simulink model "sim_battery_pack_simulink_with_EV_Load"  (R2021b)
settings: Solver=FixedStepAuto  StartTime=0.0  StopTime=3460.480  FixedStep=0.01  RelTol=1e-3
values from neighbouring files (symbols this model uses):
  Af = 1.4*1.6    (= 2.24)    [battery_pack_init_18_11.m]
  b = 0.002    [battery_pack_init_18_11.m]
  Batt_Eff = .98    (= 0.98)    [battery_pack_init_18_11.m]
  Batt_Ene_Cap = 7.37    [battery_pack_init_18_11.m]
  cd = 0.45    [battery_pack_init_18_11.m]
  dt = 0.01    [battery_pack_init_18_11.m]
  g = 9.81    [battery_pack_init_18_11.m]
  Gr = 5.75*.85    (= 4.8875)    [battery_pack_init_18_11.m]
  Grade = 7    [battery_pack_init_18_11.m]
  Ini_SOC = 100    [battery_pack_init_18_11.m]
  kappa = 0.1    [battery_pack_init_18_11.m]
  M = M_k+M_P    (= 445)    [battery_pack_init_18_11.m]
  M_Trq = T_m    [battery_pack_init_18_11.m]
  M_w = w_m    [battery_pack_init_18_11.m]
  Mot_Eff = .9    (= 0.9)    [battery_pack_init_18_11.m]
  mu = 0.016    [battery_pack_init_18_11.m]
  Np = 7    [battery_pack_init_18_11.m]
  Ns = 12    [battery_pack_init_18_11.m]
  Qgain = 1    [battery_pack_init_18_11.m]
  R0 = zeros(numpoles,1)    [battery_pack_init_18_11.m]
  R0Param = getParamESC('R0Param',T,cell_model)    [battery_pack_init_18_11.m]
  R_w = .3048/2    (= 0.1524)    [battery_pack_init_18_11.m]
  Re_spe_max = 50*5/18    (= 13.8888888889)    [battery_pack_init_18_11.m]
  Re_spe_min = 0*5/18    (= 0)    [battery_pack_init_18_11.m]
  rho = 1.225    [battery_pack_init_18_11.m]
  rt = .0008    (= 0.0008)    [battery_pack_init_18_11.m]
  T = 40    [battery_pack_init_18_11.m]
  T_MIDC = T_MIDC(1:72)    [battery_pack_init_18_11.m]
  Trans_Eff = .95    (= 0.95)    [battery_pack_init_18_11.m]
  V_MIDC = V_MIDC(1:72)    [battery_pack_init_18_11.m]
  Z0 = 0.75 + (1-0.75).*rand(1,Np)    [battery_pack_init_18_11.m]
undefined symbols (not defined in the file or in its folder): cell_model, FLbattery, gain, iload, sigbuilder_block, VMIDC
libraries: simulink x16, autolibshared x2, slpidlib x1, simulink_extras x1
(part 1 of 17)
settings Model: Creator=User  LastModifiedBy=adhip
settings SolverCC: AlgebraicLoopSolver=TrustRegion

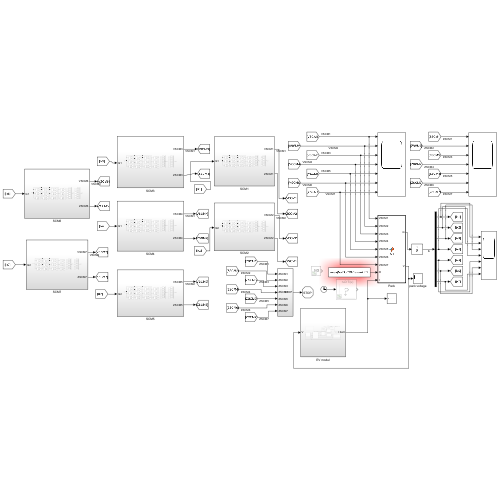
[thumbnail: Simulink's stored preview of the top-level diagram]
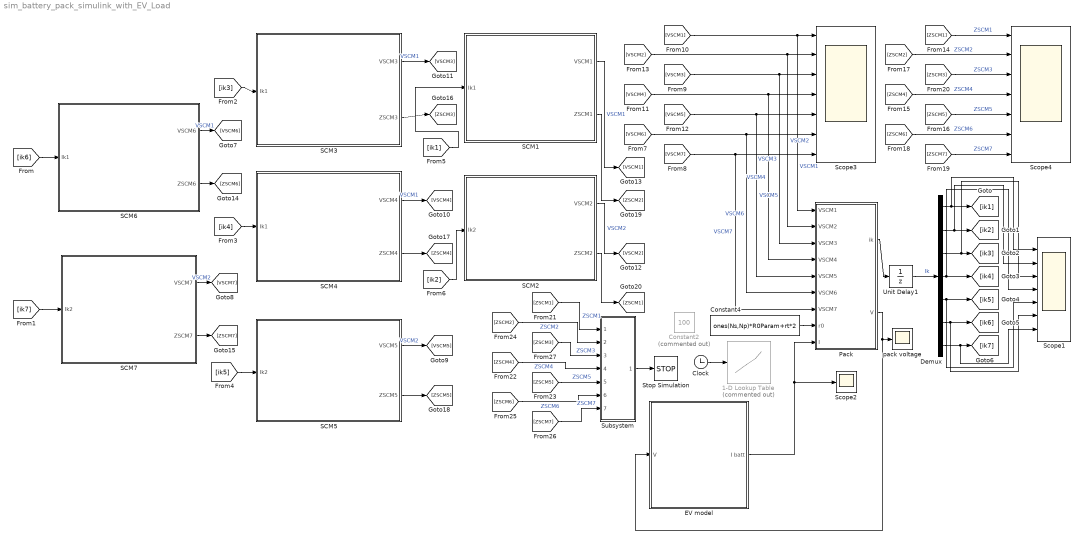
== system sim_battery_pack_simulink_with_EV_Load ==
  1-D Lookup Table : Lookup_n-D  Commented=on  NumberOfTableDimensions=1  BreakpointsForDimension1=0:0.01:3460.480  Table=iload  InternalRulePriority=Speed  RndMeth=Simplest  InputSameDT=on
  Clock : Clock
  Constant2 : Constant  Commented=on  Value=100
  Constant4 : Constant  Value=ones(Ns,Np)*R0Param+rt*2
  Demux : Demux  Outputs=7
  EV model : Subsystem
  Pack : MATLAB Function  TreatAsAtomicUnit=on
  SCM1 : Subsystem
  SCM2 : Subsystem
  SCM3 : Subsystem
  SCM4 : Subsystem
  SCM5 : Subsystem
  SCM6 : Subsystem
  SCM7 : Subsystem
  Scope1 : Scope  NumInputPorts=7
  Scope2 : Scope
  Scope3 : Scope  NumInputPorts=7
  Scope4 : Scope  NumInputPorts=7
  Stop Simulation : Stop
  Subsystem : Subsystem
  Unit Delay1 : UnitDelay  SampleTime=-1  HasFrameUpgradeWarning=on
  pack voltage : Scope
  wires:
  EV model/1(I batt) -> Pack/9(I), Scope2/1
  [VSCM1] -> Pack/1(VSCM1), Scope3/1  "VSCM1"
  [VSCM2] -> Scope3/2, Pack/2(VSCM2)  "VSCM2"
  Pack/1(ik) -> Unit Delay1/1
  Unit Delay1/1 -> Demux/1  "Ik"
  Constant4/1 -> Pack/8(r0)
  Clock/1 -> 1-D Lookup Table/1
  [VSCM3] -> Scope3/3, Pack/3(VSCM3)  "VSCM3"
  [VSCM4] -> Pack/4(VSCM4), Scope3/4  "VSCM4"
  [VSCM5] -> Pack/5(VSCM5), Scope3/5  "VSCM5"
  [VSCM6] -> Pack/6(VSCM6), Scope3/6  "VSCM6"
  [VSCM7] -> Scope3/7, Pack/7(VSCM7)  "VSCM7"
  [ik7] -> SCM7/1(Ik2)
  [ik6] -> SCM6/1(Ik1)
  [ik3] -> SCM3/1(Ik1)
  [ik4] -> SCM4/1(Ik1)
  [ik5] -> SCM5/1(Ik2)
  [ik2] -> SCM2/1(Ik2)
  [ik1] -> SCM1/1(Ik1)
  Demux/1 -> Scope1/1, [ik1]
  Demux/2 -> [ik2], Scope1/2
  Demux/3 -> Scope1/3, [ik3]
  Demux/4 -> [ik4], Scope1/4
  Demux/5 -> [ik5], Scope1/5
  Demux/6 -> [ik6], Scope1/6
  Demux/7 -> Scope1/7, [ik7]
  SCM6/1(VSCM6) -> [VSCM6]  "VSCM1"
  SCM7/1(VSCM7) -> [VSCM7]  "VSCM2"
  SCM1/1(VSCM1) -> [VSCM1]  "VSCM1"
  SCM2/1(VSCM2) -> [VSCM2]  "VSCM2"
  SCM5/1(VSCM5) -> [VSCM5]  "VSCM2"
  SCM4/1(VSCM4) -> [VSCM4]  "VSCM1"
  SCM3/1(VSCM3) -> [VSCM3]  "VSCM1"
  Pack/2(V) -> pack voltage/1, EV model/1(V)
  SCM6/2(ZSCM6) -> [ZSCM6]
  SCM7/2(ZSCM7) -> [ZSCM7]
  SCM3/2(ZSCM3) -> [ZSCM3]
  SCM4/2(ZSCM4) -> [ZSCM4]
  SCM5/2(ZSCM5) -> [ZSCM5]
  SCM1/2(ZSCM1) -> [ZSCM2]
  SCM2/2(ZSCM2) -> [ZSCM1]
  [ZSCM7] -> Scope4/7  "ZSCM7"
  [ZSCM6] -> Scope4/6  "ZSCM6"
  [ZSCM5] -> Scope4/5  "ZSCM5"
  [ZSCM4] -> Scope4/4  "ZSCM4"
  [ZSCM3] -> Scope4/3  "ZSCM3"
  [ZSCM2] -> Scope4/2  "ZSCM2"
  [ZSCM1] -> Scope4/1  "ZSCM1"
  [ZSCM2] -> Subsystem/2(ZSCM2)  "ZSCM2"
  [ZSCM4] -> Subsystem/4(ZSCM4)  "ZSCM4"
  [ZSCM6] -> Subsystem/6(ZSCM6)  "ZSCM6"
  [ZSCM1] -> Subsystem/1(ZSCM1)  "ZSCM1"
  [ZSCM3] -> Subsystem/3(ZSCM3)  "ZSCM3"
  [ZSCM5] -> Subsystem/5(ZSCM5)  "ZSCM5"
  [ZSCM7] -> Subsystem/7(ZSCM7)  "ZSCM7"
  Subsystem/1(STOP) -> Stop Simulation/1

== system sim_battery_pack_simulink_with_EV_Load/EV model ==
  V : Inport
  Battery1 : Subsystem
      settings: PortSchema="{\"entries\":[{\"content\":{\"sides\":[{\"content\":{\"connectorIds\":[\"Out4\",\"In1\"]},\"type\":\"ConnectorPlacement.EquallySpacedRectSide\",\"uuid\":\"95f9873b-fe01-4ff7-a5ab-aada3bc95a03\"},{\"content\":{\"connectorIds\":[\"Out1\",\"In2\",\"Out2\",\"Out3\"],\"side\":\"RIGHT\"},\"type\":\"ConnectorPlacement.EquallySpacedRectSide\",\"uuid\":\"b4897c1e-778c-4bc7-a7f1-163b7f4cdad4\"},{\"content\":{\"connectorIds\":[],\"side\":\"TOP\"},\"type\":\"ConnectorPlacement.EquallySpacedRectSide\",\"uuid\":\"a4f74249-cbee-46b9-95a1-ffe2d651d1aa\"}]},\"type\":\"ConnectorPlacement.EquallySpacedConnector\",\"uuid\":\"65519a53-4300-47bd-84a6-9cdab8c1658d\"}],\"packageUris\":[\"http://schema.mathworks.com/mf0/Connector/R2020b\"],\"version\":\"1.0\"}"
  Constant3 : Constant  Value=7.37
  Constant4 : Constant
  Controller : Subsystem
      settings: PortSchema="{\"entries\":[{\"content\":{\"sides\":[{\"content\":{\"connectorIds\":[\"In1\",\"In2\",\"In3\"]},\"type\":\"ConnectorPlacement.EquallySpacedRectSide\",\"uuid\":\"7181f2fb-814d-454b-bbdd-5a6429464cde\"},{\"content\":{\"connectorIds\":[\"Out1\",\"In6\",\"Out2\"],\"side\":\"RIGHT\"},\"type\":\"ConnectorPlacement.EquallySpacedRectSide\",\"uuid\":\"9f09df5c-a21b-4dbe-b9f4-fd639a3fc7b6\"},{\"content\":{\"connectorIds\":[\"In4\",\"In5\"],\"side\":\"TOP\"},\"type\":\"ConnectorPlacement.EquallySpacedRectSide\",\"uuid\":\"cea066f6-5d29-4bfe-a52b-88d077042081\"}]},\"type\":\"ConnectorPlacement.EquallySpacedConnector\",\"uuid\":\"89d9cb73-964c-472c-86a0-f36e993decee\"}],\"packageUris\":[\"http://schema.mathworks.com/mf0/Connector/R2020b\"],\"version\":\"1.0\"}"
  Display2 : Display
  Divide : Product  Inputs=*/
  Driver : Subsystem
  Motor : Subsystem
  Product1 : Product
  Scope : Scope
  Scope1 : Scope  NumInputPorts=2
  Subtract : Sum  Inputs=+-
  Transmission : Subsystem
      settings: PortSchema="{\"entries\":[{\"content\":{\"sides\":[{\"content\":{\"connectorIds\":[\"In1\",\"Out2\"]},\"type\":\"ConnectorPlacement.EquallySpacedRectSide\",\"uuid\":\"6a60ea79-1d6a-43be-8c6e-faa96b9426ae\"},{\"content\":{\"connectorIds\":[\"Out1\",\"In2\"],\"side\":\"RIGHT\"},\"type\":\"ConnectorPlacement.EquallySpacedRectSide\",\"uuid\":\"ce7e119a-d2f4-42be-b472-f935cef86375\"},{\"content\":{\"connectorIds\":[],\"side\":\"TOP\"},\"type\":\"ConnectorPlacement.EquallySpacedRectSide\",\"uuid\":\"7967fcd3-5be4-4a26-8ccb-3cce446b495a\"}]},\"type\":\"ConnectorPlacement.EquallySpacedConnector\",\"uuid\":\"10659099-893a-4c78-98f4-a4e8ec8b982a\"}],\"packageUris\":[\"http://schema.mathworks.com/mf0/Connector/R2020b\"],\"version\":\"1.0\"}"
  Vehicle Dynamics : Subsystem
      settings: PortSchema="{\"entries\":[{\"content\":{\"sides\":[{\"content\":{\"connectorIds\":[\"In1\",\"Out3\",\"Out4\",\"In2\"]},\"type\":\"ConnectorPlacement.EquallySpacedRectSide\",\"uuid\":\"6a60ea79-1d6a-43be-8c6e-faa96b9426ae\"},{\"content\":{\"connectorIds\":[\"Out1\"],\"side\":\"RIGHT\"},\"type\":\"ConnectorPlacement.EquallySpacedRectSide\",\"uuid\":\"ce7e119a-d2f4-42be-b472-f935cef86375\"},{\"content\":{\"connectorIds\":[\"Out2\"],\"side\":\"TOP\"},\"type\":\"ConnectorPlacement.EquallySpacedRectSide\",\"uuid\":\"7967fcd3-5be4-4a26-8ccb-3cce446b495a\"}]},\"type\":\"ConnectorPlacement.EquallySpacedConnector\",\"uuid\":\"10659099-893a-4c78-98f4-a4e8ec8b982a\"}],\"packageUris\":[\"http://schema.mathworks.com/mf0/Connector/R2020b\"],\"version\":\"1.0\"}"
  Vehicle Monitoring : Subsystem  Commented=on
  km : Display
  kwhr/km : Display
  I batt : Outport
  tag scope: Soc=global
  wires:
  Product1/1 -> Divide/1
  Battery1/1(SOC) -> [Soc], Scope/1, Display2/1, Subtract/2
  Controller/1(TrqCmd) -> Motor/1(TrqCmd)
  Subtract/1 -> Product1/2
  Constant4/1 -> Subtract/1
  Motor/2(Mtr_trq) -> Transmission/1(MtrTrq)
  Vehicle Dynamics/4(VKm/h) -> Scope1/2
  Battery1/3(Regen_Pow_Lim) -> Controller/5(Regen_Lim)
  Divide/1 -> kwhr/km/1
  Driver/3(Vref) -> Scope1/1
  Driver/2(DecelCmd) -> Controller/2(Brake)
  Motor/1(Batt_Pow_Cons) -> Battery1/1(Battery power)
  Vehicle Dynamics/2(Dis) -> Divide/2, km/1
  Vehicle Dynamics/1(VehSpd) -> Controller/3(VehSpd), Driver/1(VelFdbk)
  Battery1/2(Draw_Pow_Lim) -> Controller/4(Draw_Lim)
  Transmission/1(AxleTrq) -> Vehicle Dynamics/1(AxleTrq)
  Controller/2(BrkForce) -> Vehicle Dynamics/2(BrakeForce)
  Driver/1(AccelCmd) -> Controller/1(AccelCmd)
  Transmission/2(MtrSpd) -> Controller/6(MtrSpd), Motor/2(MtrSpd)
  Vehicle Dynamics/3(AxleSpd) -> Transmission/2(AxleSpd)
  Constant3/1 -> Product1/1
  Battery1/4(I batt) -> I batt/1
  V/1 -> Battery1/2(V)

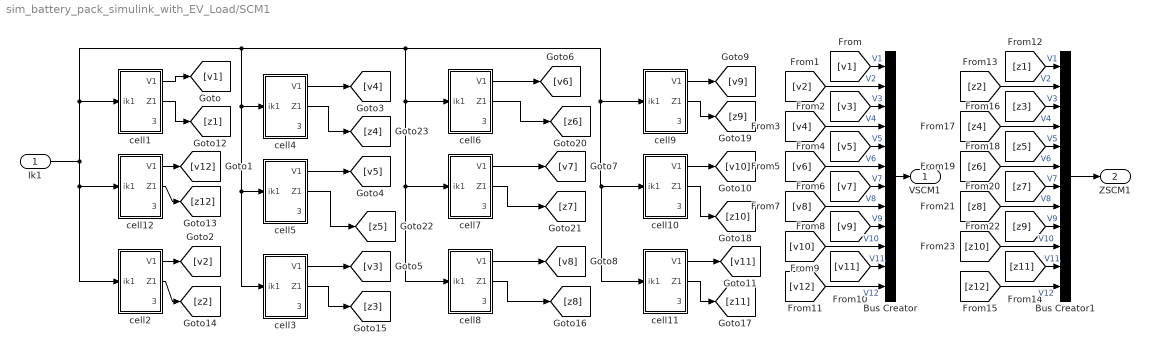
== system sim_battery_pack_simulink_with_EV_Load/SCM1 ==
  Ik1 : Inport
  Bus Creator : BusCreator  Inputs=12
  Bus Creator1 : BusCreator  Inputs=12
  cell1 : Subsystem
  cell10 : Subsystem
  cell11 : Subsystem
  cell12 : Subsystem
  cell2 : Subsystem
  cell3 : Subsystem
  cell4 : Subsystem
  cell5 : Subsystem
  cell6 : Subsystem
  cell7 : Subsystem
  cell8 : Subsystem
  cell9 : Subsystem
  VSCM1 : Outport
  ZSCM1 : Outport  Port=2
  wires:
  cell11/1(V1) -> [v11]
  cell8/1(V1) -> [v8]
  cell2/1(V1) -> [v2]
  cell1/1(V1) -> [v1]
  cell12/1(V1) -> [v12]
  cell7/1(V1) -> [v7]
  cell10/1(V1) -> [v10]
  Ik1/1 -> cell2/1(ik1), cell12/1(ik1), cell1/1(ik1), cell9/1(ik1), cell11/1(ik1), cell10/1(ik1), cell6/1(ik1), cell8/1(ik1), cell7/1(ik1), cell4/1(ik1), cell5/1(ik1), cell3/1(ik1)
  [v1] -> Bus Creator/1  "V1"
  [v2] -> Bus Creator/2  "V2"
  cell4/1(V1) -> [v4]
  cell5/1(V1) -> [v5]
  cell3/1(V1) -> [v3]
  cell6/1(V1) -> [v6]
  cell9/1(V1) -> [v9]
  [v3] -> Bus Creator/3  "V3"
  [v4] -> Bus Creator/4  "V4"
  [v5] -> Bus Creator/5  "V5"
  [v6] -> Bus Creator/6  "V6"
  [v7] -> Bus Creator/7  "V7"
  [v8] -> Bus Creator/8  "V8"
  [v9] -> Bus Creator/9  "V9"
  [v10] -> Bus Creator/10  "V10"
  [v11] -> Bus Creator/11  "V11"
  [v12] -> Bus Creator/12  "V12"
  Bus Creator/1 -> VSCM1/1
  cell1/2(Z1) -> [z1]
  cell12/2(Z1) -> [z12]
  cell2/2(Z1) -> [z2]
  cell8/2(Z1) -> [z8]
  cell11/2(Z1) -> [z11]
  cell10/2(Z1) -> [z10]
  cell9/2(Z1) -> [z9]
  cell6/2(Z1) -> [z6]
  cell7/2(Z1) -> [z7]
  cell3/2(Z1) -> [z3]
  cell5/2(Z1) -> [z5]
  cell4/2(Z1) -> [z4]
  Bus Creator1/1 -> ZSCM1/1
  [z12] -> Bus Creator1/12  "V12"
  [z11] -> Bus Creator1/11  "V11"
  [z10] -> Bus Creator1/10  "V10"
  [z9] -> Bus Creator1/9  "V9"
  [z8] -> Bus Creator1/8  "V8"
  [z7] -> Bus Creator1/7  "V7"
  [z6] -> Bus Creator1/6  "V6"
  [z5] -> Bus Creator1/5  "V5"
  [z4] -> Bus Creator1/4  "V4"
  [z3] -> Bus Creator1/3  "V3"
  [z2] -> Bus Creator1/2  "V2"
  [z1] -> Bus Creator1/1  "V1"

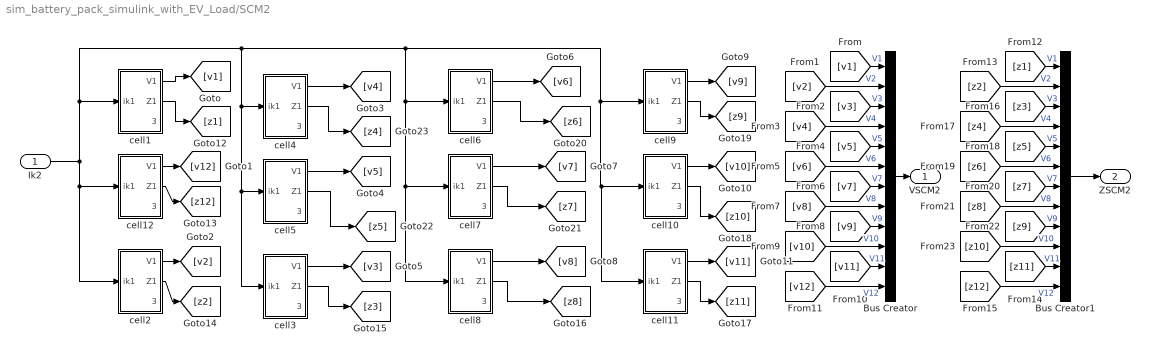
== system sim_battery_pack_simulink_with_EV_Load/SCM2 ==
  Ik2 : Inport
  Bus Creator : BusCreator  Inputs=12
  Bus Creator1 : BusCreator  Inputs=12
  cell1 : Subsystem
  cell10 : Subsystem
  cell11 : Subsystem
  cell12 : Subsystem
  cell2 : Subsystem
  cell3 : Subsystem
  cell4 : Subsystem
  cell5 : Subsystem
  cell6 : Subsystem
  cell7 : Subsystem
  cell8 : Subsystem
  cell9 : Subsystem
  VSCM2 : Outport
  ZSCM2 : Outport  Port=2
  wires:
  [z1] -> Bus Creator1/1  "V1"
  [z2] -> Bus Creator1/2  "V2"
  [z3] -> Bus Creator1/3  "V3"
  [z4] -> Bus Creator1/4  "V4"
  [z5] -> Bus Creator1/5  "V5"
  [z6] -> Bus Creator1/6  "V6"
  [z7] -> Bus Creator1/7  "V7"
  [z8] -> Bus Creator1/8  "V8"
  [z9] -> Bus Creator1/9  "V9"
  [z10] -> Bus Creator1/10  "V10"
  [z11] -> Bus Creator1/11  "V11"
  [z12] -> Bus Creator1/12  "V12"
  Bus Creator1/1 -> ZSCM2/1
  cell4/2(Z1) -> [z4]
  cell5/2(Z1) -> [z5]
  cell3/2(Z1) -> [z3]
  cell7/2(Z1) -> [z7]
  cell6/2(Z1) -> [z6]
  cell9/2(Z1) -> [z9]
  cell10/2(Z1) -> [z10]
  cell11/2(Z1) -> [z11]
  cell8/2(Z1) -> [z8]
  cell2/2(Z1) -> [z2]
  cell12/2(Z1) -> [z12]
  cell1/2(Z1) -> [z1]
  Bus Creator/1 -> VSCM2/1
  [v12] -> Bus Creator/12  "V12"
  [v11] -> Bus Creator/11  "V11"
  [v10] -> Bus Creator/10  "V10"
  [v9] -> Bus Creator/9  "V9"
  [v8] -> Bus Creator/8  "V8"
  [v7] -> Bus Creator/7  "V7"
  [v6] -> Bus Creator/6  "V6"
  [v5] -> Bus Creator/5  "V5"
  [v4] -> Bus Creator/4  "V4"
  [v3] -> Bus Creator/3  "V3"
  cell9/1(V1) -> [v9]
  cell6/1(V1) -> [v6]
  cell3/1(V1) -> [v3]
  cell5/1(V1) -> [v5]
  cell4/1(V1) -> [v4]
  [v2] -> Bus Creator/2  "V2"
  [v1] -> Bus Creator/1  "V1"
  Ik2/1 -> cell3/1(ik1), cell5/1(ik1), cell4/1(ik1), cell7/1(ik1), cell8/1(ik1), cell6/1(ik1), cell10/1(ik1), cell11/1(ik1), cell9/1(ik1), cell1/1(ik1), cell12/1(ik1), cell2/1(ik1)
  cell10/1(V1) -> [v10]
  cell7/1(V1) -> [v7]
  cell12/1(V1) -> [v12]
  cell1/1(V1) -> [v1]
  cell2/1(V1) -> [v2]
  cell8/1(V1) -> [v8]
  cell11/1(V1) -> [v11]

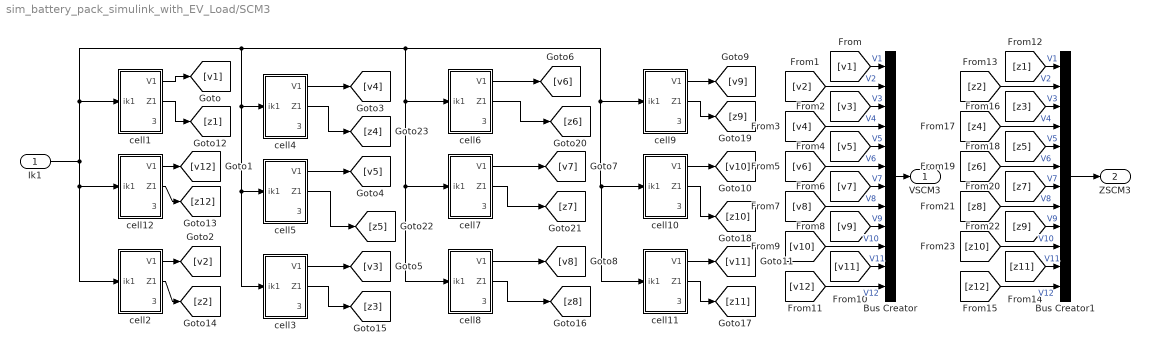
== system sim_battery_pack_simulink_with_EV_Load/SCM3 ==
  Ik1 : Inport
  Bus Creator : BusCreator  Inputs=12
  Bus Creator1 : BusCreator  Inputs=12
  cell1 : Subsystem
  cell10 : Subsystem
  cell11 : Subsystem
  cell12 : Subsystem
  cell2 : Subsystem
  cell3 : Subsystem
  cell4 : Subsystem
  cell5 : Subsystem
  cell6 : Subsystem
  cell7 : Subsystem
  cell8 : Subsystem
  cell9 : Subsystem
  VSCM3 : Outport
  ZSCM3 : Outport  Port=2
  wires:
  cell11/1(V1) -> [v11]
  cell8/1(V1) -> [v8]
  cell2/1(V1) -> [v2]
  cell1/1(V1) -> [v1]
  cell12/1(V1) -> [v12]
  cell7/1(V1) -> [v7]
  cell10/1(V1) -> [v10]
  Ik1/1 -> cell2/1(ik1), cell12/1(ik1), cell1/1(ik1), cell9/1(ik1), cell11/1(ik1), cell10/1(ik1), cell6/1(ik1), cell8/1(ik1), cell7/1(ik1), cell4/1(ik1), cell5/1(ik1), cell3/1(ik1)
  [v1] -> Bus Creator/1  "V1"
  [v2] -> Bus Creator/2  "V2"
  cell4/1(V1) -> [v4]
  cell5/1(V1) -> [v5]
  cell3/1(V1) -> [v3]
  cell6/1(V1) -> [v6]
  cell9/1(V1) -> [v9]
  [v3] -> Bus Creator/3  "V3"
  [v4] -> Bus Creator/4  "V4"
  [v5] -> Bus Creator/5  "V5"
  [v6] -> Bus Creator/6  "V6"
  [v7] -> Bus Creator/7  "V7"
  [v8] -> Bus Creator/8  "V8"
  [v9] -> Bus Creator/9  "V9"
  [v10] -> Bus Creator/10  "V10"
  [v11] -> Bus Creator/11  "V11"
  [v12] -> Bus Creator/12  "V12"
  Bus Creator/1 -> VSCM3/1
  cell1/2(Z1) -> [z1]
  cell12/2(Z1) -> [z12]
  cell2/2(Z1) -> [z2]
  cell8/2(Z1) -> [z8]
  cell11/2(Z1) -> [z11]
  cell10/2(Z1) -> [z10]
  cell9/2(Z1) -> [z9]
  cell6/2(Z1) -> [z6]
  cell7/2(Z1) -> [z7]
  cell3/2(Z1) -> [z3]
  cell5/2(Z1) -> [z5]
  cell4/2(Z1) -> [z4]
  Bus Creator1/1 -> ZSCM3/1
  [z12] -> Bus Creator1/12  "V12"
  [z11] -> Bus Creator1/11  "V11"
  [z10] -> Bus Creator1/10  "V10"
  [z9] -> Bus Creator1/9  "V9"
  [z8] -> Bus Creator1/8  "V8"
  [z7] -> Bus Creator1/7  "V7"
  [z6] -> Bus Creator1/6  "V6"
  [z5] -> Bus Creator1/5  "V5"
  [z4] -> Bus Creator1/4  "V4"
  [z3] -> Bus Creator1/3  "V3"
  [z2] -> Bus Creator1/2  "V2"
  [z1] -> Bus Creator1/1  "V1"

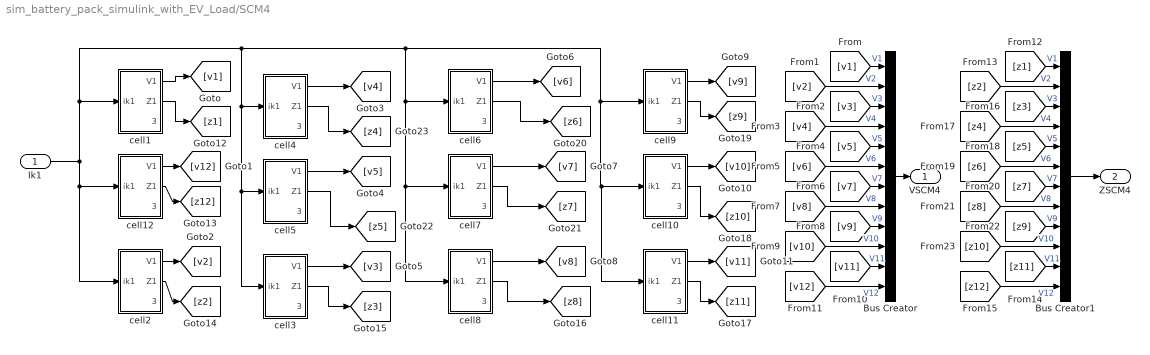
== system sim_battery_pack_simulink_with_EV_Load/SCM4 ==
  Ik1 : Inport
  Bus Creator : BusCreator  Inputs=12
  Bus Creator1 : BusCreator  Inputs=12
  cell1 : Subsystem
  cell10 : Subsystem
  cell11 : Subsystem
  cell12 : Subsystem
  cell2 : Subsystem
  cell3 : Subsystem
  cell4 : Subsystem
  cell5 : Subsystem
  cell6 : Subsystem
  cell7 : Subsystem
  cell8 : Subsystem
  cell9 : Subsystem
  VSCM4 : Outport
  ZSCM4 : Outport  Port=2
  wires:
  [z1] -> Bus Creator1/1  "V1"
  [z2] -> Bus Creator1/2  "V2"
  [z3] -> Bus Creator1/3  "V3"
  [z4] -> Bus Creator1/4  "V4"
  [z5] -> Bus Creator1/5  "V5"
  [z6] -> Bus Creator1/6  "V6"
  [z7] -> Bus Creator1/7  "V7"
  [z8] -> Bus Creator1/8  "V8"
  [z9] -> Bus Creator1/9  "V9"
  [z10] -> Bus Creator1/10  "V10"
  [z11] -> Bus Creator1/11  "V11"
  [z12] -> Bus Creator1/12  "V12"
  Bus Creator1/1 -> ZSCM4/1
  cell4/2(Z1) -> [z4]
  cell5/2(Z1) -> [z5]
  cell3/2(Z1) -> [z3]
  cell7/2(Z1) -> [z7]
  cell6/2(Z1) -> [z6]
  cell9/2(Z1) -> [z9]
  cell10/2(Z1) -> [z10]
  cell11/2(Z1) -> [z11]
  cell8/2(Z1) -> [z8]
  cell2/2(Z1) -> [z2]
  cell12/2(Z1) -> [z12]
  cell1/2(Z1) -> [z1]
  Bus Creator/1 -> VSCM4/1
  [v12] -> Bus Creator/12  "V12"
  [v11] -> Bus Creator/11  "V11"
  [v10] -> Bus Creator/10  "V10"
  [v9] -> Bus Creator/9  "V9"
  [v8] -> Bus Creator/8  "V8"
  [v7] -> Bus Creator/7  "V7"
  [v6] -> Bus Creator/6  "V6"
  [v5] -> Bus Creator/5  "V5"
  [v4] -> Bus Creator/4  "V4"
  [v3] -> Bus Creator/3  "V3"
  cell9/1(V1) -> [v9]
  cell6/1(V1) -> [v6]
  cell3/1(V1) -> [v3]
  cell5/1(V1) -> [v5]
  cell4/1(V1) -> [v4]
  [v2] -> Bus Creator/2  "V2"
  [v1] -> Bus Creator/1  "V1"
  Ik1/1 -> cell3/1(ik1), cell5/1(ik1), cell4/1(ik1), cell7/1(ik1), cell8/1(ik1), cell6/1(ik1), cell10/1(ik1), cell11/1(ik1), cell9/1(ik1), cell1/1(ik1), cell12/1(ik1), cell2/1(ik1)
  cell10/1(V1) -> [v10]
  cell7/1(V1) -> [v7]
  cell12/1(V1) -> [v12]
  cell1/1(V1) -> [v1]
  cell2/1(V1) -> [v2]
  cell8/1(V1) -> [v8]
  cell11/1(V1) -> [v11]

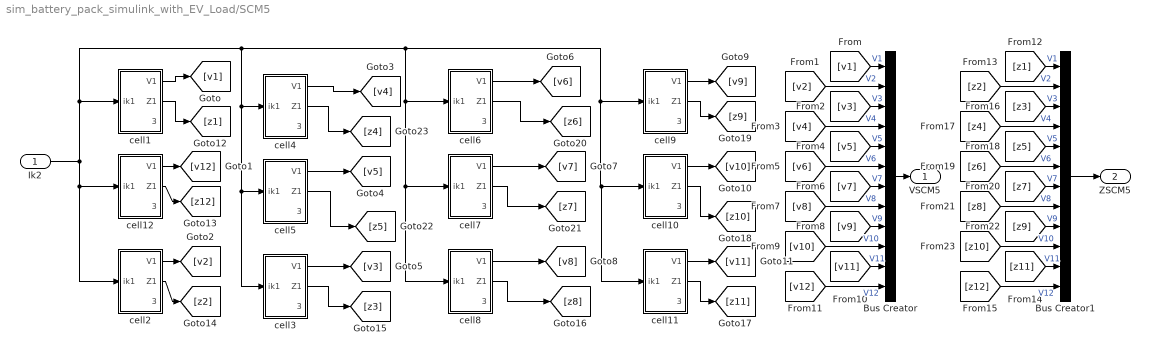
== system sim_battery_pack_simulink_with_EV_Load/SCM5 ==
  Ik2 : Inport
  Bus Creator : BusCreator  Inputs=12
  Bus Creator1 : BusCreator  Inputs=12
  cell1 : Subsystem
  cell10 : Subsystem
  cell11 : Subsystem
  cell12 : Subsystem
  cell2 : Subsystem
  cell3 : Subsystem
  cell4 : Subsystem
  cell5 : Subsystem
  cell6 : Subsystem
  cell7 : Subsystem
  cell8 : Subsystem
  cell9 : Subsystem
  VSCM5 : Outport
  ZSCM5 : Outport  Port=2
  wires:
  [z1] -> Bus Creator1/1  "V1"
  [z2] -> Bus Creator1/2  "V2"
  [z3] -> Bus Creator1/3  "V3"
  [z4] -> Bus Creator1/4  "V4"
  [z5] -> Bus Creator1/5  "V5"
  [z6] -> Bus Creator1/6  "V6"
  [z7] -> Bus Creator1/7  "V7"
  [z8] -> Bus Creator1/8  "V8"
  [z9] -> Bus Creator1/9  "V9"
  [z10] -> Bus Creator1/10  "V10"
  [z11] -> Bus Creator1/11  "V11"
  [z12] -> Bus Creator1/12  "V12"
  Bus Creator1/1 -> ZSCM5/1
  cell4/2(Z1) -> [z4]
  cell5/2(Z1) -> [z5]
  cell3/2(Z1) -> [z3]
  cell7/2(Z1) -> [z7]
  cell6/2(Z1) -> [z6]
  cell9/2(Z1) -> [z9]
  cell10/2(Z1) -> [z10]
  cell11/2(Z1) -> [z11]
  cell8/2(Z1) -> [z8]
  cell2/2(Z1) -> [z2]
  cell12/2(Z1) -> [z12]
  cell1/2(Z1) -> [z1]
  Bus Creator/1 -> VSCM5/1
  [v12] -> Bus Creator/12  "V12"
  [v11] -> Bus Creator/11  "V11"
  [v10] -> Bus Creator/10  "V10"
  [v9] -> Bus Creator/9  "V9"
  [v8] -> Bus Creator/8  "V8"
  [v7] -> Bus Creator/7  "V7"
  [v6] -> Bus Creator/6  "V6"
  [v5] -> Bus Creator/5  "V5"
  [v4] -> Bus Creator/4  "V4"
  [v3] -> Bus Creator/3  "V3"
  cell9/1(V1) -> [v9]
  cell6/1(V1) -> [v6]
  cell3/1(V1) -> [v3]
  cell5/1(V1) -> [v5]
  cell4/1(V1) -> [v4]
  [v2] -> Bus Creator/2  "V2"
  [v1] -> Bus Creator/1  "V1"
  Ik2/1 -> cell3/1(ik1), cell5/1(ik1), cell4/1(ik1), cell7/1(ik1), cell8/1(ik1), cell6/1(ik1), cell10/1(ik1), cell11/1(ik1), cell9/1(ik1), cell1/1(ik1), cell12/1(ik1), cell2/1(ik1)
  cell10/1(V1) -> [v10]
  cell7/1(V1) -> [v7]
  cell12/1(V1) -> [v12]
  cell1/1(V1) -> [v1]
  cell2/1(V1) -> [v2]
  cell8/1(V1) -> [v8]
  cell11/1(V1) -> [v11]

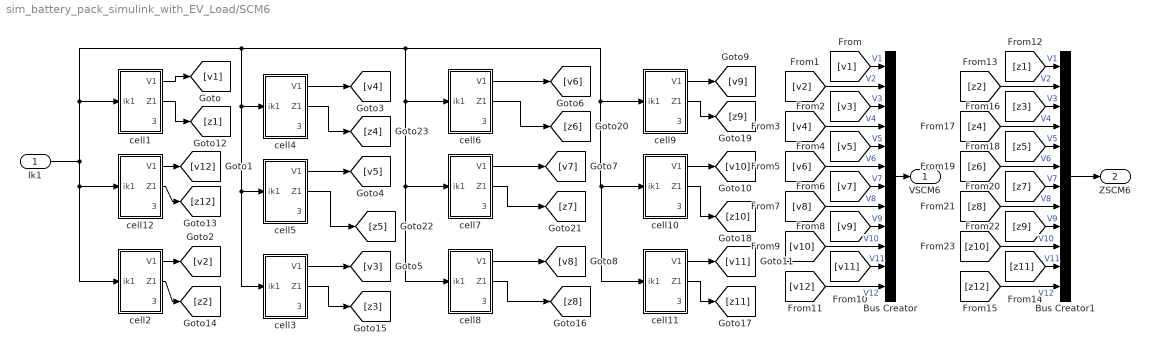
== system sim_battery_pack_simulink_with_EV_Load/SCM6 ==
  Ik1 : Inport
  Bus Creator : BusCreator  Inputs=12
  Bus Creator1 : BusCreator  Inputs=12
  cell1 : Subsystem
  cell10 : Subsystem
  cell11 : Subsystem
  cell12 : Subsystem
  cell2 : Subsystem
  cell3 : Subsystem
  cell4 : Subsystem
  cell5 : Subsystem
  cell6 : Subsystem
  cell7 : Subsystem
  cell8 : Subsystem
  cell9 : Subsystem
  VSCM6 : Outport
  ZSCM6 : Outport  Port=2
  wires:
  [z1] -> Bus Creator1/1  "V1"
  [z2] -> Bus Creator1/2  "V2"
  [z3] -> Bus Creator1/3  "V3"
  [z4] -> Bus Creator1/4  "V4"
  [z5] -> Bus Creator1/5  "V5"
  [z6] -> Bus Creator1/6  "V6"
  [z7] -> Bus Creator1/7  "V7"
  [z8] -> Bus Creator1/8  "V8"
  [z9] -> Bus Creator1/9  "V9"
  [z10] -> Bus Creator1/10  "V10"
  [z11] -> Bus Creator1/11  "V11"
  [z12] -> Bus Creator1/12  "V12"
  Bus Creator1/1 -> ZSCM6/1
  cell4/2(Z1) -> [z4]
  cell5/2(Z1) -> [z5]
  cell3/2(Z1) -> [z3]
  cell7/2(Z1) -> [z7]
  cell6/2(Z1) -> [z6]
  cell9/2(Z1) -> [z9]
  cell10/2(Z1) -> [z10]
  cell11/2(Z1) -> [z11]
  cell8/2(Z1) -> [z8]
  cell2/2(Z1) -> [z2]
  cell12/2(Z1) -> [z12]
  cell1/2(Z1) -> [z1]
  Bus Creator/1 -> VSCM6/1
  [v12] -> Bus Creator/12  "V12"
  [v11] -> Bus Creator/11  "V11"
  [v10] -> Bus Creator/10  "V10"
  [v9] -> Bus Creator/9  "V9"
  [v8] -> Bus Creator/8  "V8"
  [v7] -> Bus Creator/7  "V7"
  [v6] -> Bus Creator/6  "V6"
  [v5] -> Bus Creator/5  "V5"
  [v4] -> Bus Creator/4  "V4"
  [v3] -> Bus Creator/3  "V3"
  cell9/1(V1) -> [v9]
  cell6/1(V1) -> [v6]
  cell3/1(V1) -> [v3]
  cell5/1(V1) -> [v5]
  cell4/1(V1) -> [v4]
  [v2] -> Bus Creator/2  "V2"
  [v1] -> Bus Creator/1  "V1"
  Ik1/1 -> cell3/1(ik1), cell5/1(ik1), cell4/1(ik1), cell7/1(ik1), cell8/1(ik1), cell6/1(ik1), cell10/1(ik1), cell11/1(ik1), cell9/1(ik1), cell1/1(ik1), cell12/1(ik1), cell2/1(ik1)
  cell10/1(V1) -> [v10]
  cell7/1(V1) -> [v7]
  cell12/1(V1) -> [v12]
  cell1/1(V1) -> [v1]
  cell2/1(V1) -> [v2]
  cell8/1(V1) -> [v8]
  cell11/1(V1) -> [v11]

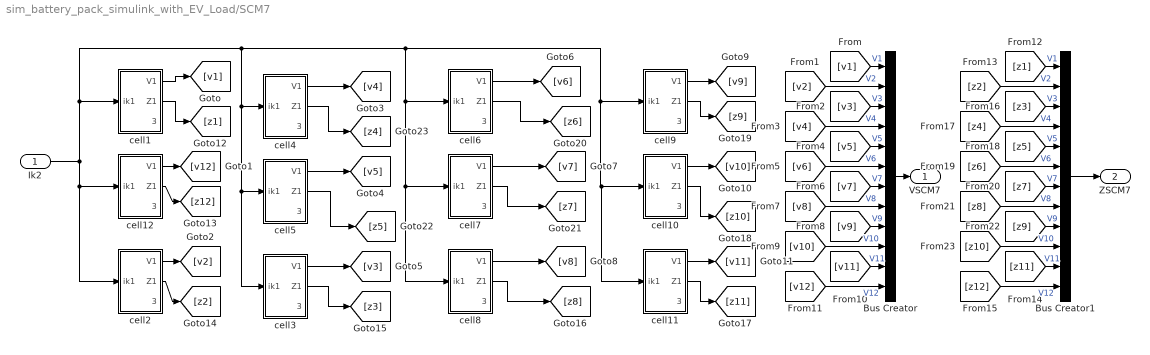
== system sim_battery_pack_simulink_with_EV_Load/SCM7 ==
  Ik2 : Inport
  Bus Creator : BusCreator  Inputs=12
  Bus Creator1 : BusCreator  Inputs=12
  cell1 : Subsystem
  cell10 : Subsystem
  cell11 : Subsystem
  cell12 : Subsystem
  cell2 : Subsystem
  cell3 : Subsystem
  cell4 : Subsystem
  cell5 : Subsystem
  cell6 : Subsystem
  cell7 : Subsystem
  cell8 : Subsystem
  cell9 : Subsystem
  VSCM7 : Outport
  ZSCM7 : Outport  Port=2
  wires:
  cell11/1(V1) -> [v11]
  cell8/1(V1) -> [v8]
  cell2/1(V1) -> [v2]
  cell1/1(V1) -> [v1]
  cell12/1(V1) -> [v12]
  cell7/1(V1) -> [v7]
  cell10/1(V1) -> [v10]
  Ik2/1 -> cell2/1(ik1), cell12/1(ik1), cell1/1(ik1), cell9/1(ik1), cell11/1(ik1), cell10/1(ik1), cell6/1(ik1), cell8/1(ik1), cell7/1(ik1), cell4/1(ik1), cell5/1(ik1), cell3/1(ik1)
  [v1] -> Bus Creator/1  "V1"
  [v2] -> Bus Creator/2  "V2"
  cell4/1(V1) -> [v4]
  cell5/1(V1) -> [v5]
  cell3/1(V1) -> [v3]
  cell6/1(V1) -> [v6]
  cell9/1(V1) -> [v9]
  [v3] -> Bus Creator/3  "V3"
  [v4] -> Bus Creator/4  "V4"
  [v5] -> Bus Creator/5  "V5"
  [v6] -> Bus Creator/6  "V6"
  [v7] -> Bus Creator/7  "V7"
  [v8] -> Bus Creator/8  "V8"
  [v9] -> Bus Creator/9  "V9"
  [v10] -> Bus Creator/10  "V10"
  [v11] -> Bus Creator/11  "V11"
  [v12] -> Bus Creator/12  "V12"
  Bus Creator/1 -> VSCM7/1
  cell1/2(Z1) -> [z1]
  cell12/2(Z1) -> [z12]
  cell2/2(Z1) -> [z2]
  cell8/2(Z1) -> [z8]
  cell11/2(Z1) -> [z11]
  cell10/2(Z1) -> [z10]
  cell9/2(Z1) -> [z9]
  cell6/2(Z1) -> [z6]
  cell7/2(Z1) -> [z7]
  cell3/2(Z1) -> [z3]
  cell5/2(Z1) -> [z5]
  cell4/2(Z1) -> [z4]
  Bus Creator1/1 -> ZSCM7/1
  [z12] -> Bus Creator1/12  "V12"
  [z11] -> Bus Creator1/11  "V11"
  [z10] -> Bus Creator1/10  "V10"
  [z9] -> Bus Creator1/9  "V9"
  [z8] -> Bus Creator1/8  "V8"
  [z7] -> Bus Creator1/7  "V7"
  [z6] -> Bus Creator1/6  "V6"
  [z5] -> Bus Creator1/5  "V5"
  [z4] -> Bus Creator1/4  "V4"
  [z3] -> Bus Creator1/3  "V3"
  [z2] -> Bus Creator1/2  "V2"
  [z1] -> Bus Creator1/1  "V1"

== system sim_battery_pack_simulink_with_EV_Load/Subsystem ==
  ZSCM1 : Inport
  ZSCM2 : Inport  Port=2
  ZSCM3 : Inport  Port=3
  ZSCM4 : Inport  Port=4
  ZSCM5 : Inport  Port=5
  ZSCM6 : Inport  Port=6
  ZSCM7 : Inport  Port=7
  Bus Creator : BusCreator  Inputs=7
  Compare To Constant : simulink/Logic and Bit Operations/Compare To Constant  relop=<=  const=0.05  OutDataTypeStr=boolean
  Display : Display
  Min of Elements : MinMax
  STOP : Outport
  wires:
  ZSCM1/1 -> Bus Creator/1
  ZSCM2/1 -> Bus Creator/2
  ZSCM3/1 -> Bus Creator/3
  ZSCM4/1 -> Bus Creator/4
  ZSCM5/1 -> Bus Creator/5
  ZSCM6/1 -> Bus Creator/6
  ZSCM7/1 -> Bus Creator/7
  Bus Creator/1 -> Display/1, Min of Elements/1
  Min of Elements/1 -> Compare To Constant/1
  Compare To Constant/1 -> STOP/1

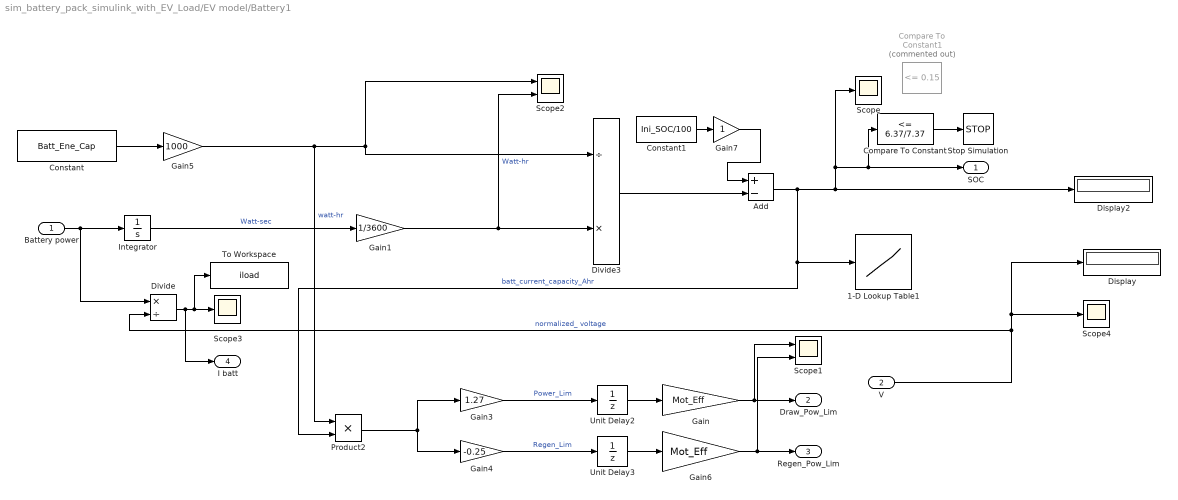
== system sim_battery_pack_simulink_with_EV_Load/EV model/Battery1 ==
  Battery power : Inport
  V : Inport  Port=2
  1-D Lookup Table1 : Lookup_n-D  NumberOfTableDimensions=1  BreakpointsForDimension1=[0,0.01,0.02,0.03,0.04,0.05,0.06,0.07,0.08,0.09,0.1,0.11,0.12,0.13,0.14,0.15,0.16,0.17,0.18,0.19,0.2,0.21,0.22,0.23,0.24,0.25,0.26,0.27,0.28,0.29,0.3,0.31,0.32,0.33,0.34,0.35,0.36,0.37,0.38,0.39,0.4,0.41,0.42,0.43,0.44,0.45,0.46,0.47,0.48,0.49,0.5,0.51,0.52,0.53,0.54,0.55,0.56,0.57,0.58,0.59,0.6,0.61,0.62,0.63,0.64,0.65,0.66,0.67,0.68,0.69,0.7,0.71,0.72,0.73,0.74,0.75,0.76,0.77,0.78,0.79,0.8,0.81,0.82,0.83,0.84,0.85,0.86,0.87,0.88,0.89,0.9,0.91,0.92,0.93,0.94,0.95,0.96,0.97,0.98,0.99,1]  Table=[31.919999999999998,36.799200000000006,37.437599999999996,38.315400000000004,38.8512,39.0678,39.5808,39.6378,39.8202,39.9456,40.0824,40.2192,40.3218,40.3195,40.5751,40.5112,40.5751,40.766400000000004,40.8918,40.9146,41.0224,41.04,41.1312,41.153999999999996,41.2224,41.256600000000006,41.3364,41.4048,41.461800000000004,41.496,41.5974,41.5644,41.6328,41.667,41.7012,41.7354,41.769600000000004,41.815200000000004,41.8722,41.9292,41.952000000000005,41.9634,42.0204,42.088800000000006,42.1686,42.2028,42.237,42.294000000000004,42.3738,42.4422,42.4992,42.6837,42.579,42.6198,42.738600000000005,42.807,42.875400000000006,42.9552,43.0122,43.092,43.1949,43.297200000000004,43.297200000000004,43.479600000000005,43.525200000000005,43.605000000000004,43.787400000000005,43.8444,43.947,44.0382,44.1978,44.289,44.391600000000004,44.5398,44.6766,44.756400000000006,44.859,44.961600000000004,45.0756,45.1896,45.3036,45.4632,45.577200000000005,45.759600000000006,45.9306,45.9876,46.135799999999996,46.34100000000001,46.443599999999996,46.580400000000004,46.7058,47.0934,47.03640000000001,47.1732,47.31,47.652,47.583600000000004,47.73180000000001,47.9598,48.2334,48.119400000000006]  ExtrapMethod=Clip  UseLastTableValue=on  InternalRulePriority=Speed  RndMeth=Simplest  InputSameDT=on
  Add : Sum  Inputs=+-
  Compare To Constant : simulink/Logic and Bit Operations/Compare To Constant  relop=<=  const=6.37/7.37  OutDataTypeStr=boolean
  Compare To Constant1 : simulink/Logic and Bit Operations/Compare To Constant  Commented=on  relop=<=  const=0.15  OutDataTypeStr=boolean
  Constant : Constant  Value=Batt_Ene_Cap
  Constant1 : Constant  Value=Ini_SOC/100
  Display : Display
  Display2 : Display
  Divide : Product  Inputs=*/
  Divide3 : Product  Inputs=/*
  Gain : Gain  Gain=Mot_Eff
  Gain1 : Gain  Gain=1/3600
  Gain3 : Gain  Gain=1.27
  Gain4 : Gain  Gain=-0.25
  Gain5 : Gain  Gain=1000
  Gain6 : Gain  Gain=Mot_Eff
  Gain7 : Gain
  Integrator : Integrator
  Product2 : Product
  Scope : Scope
  Scope1 : Scope  NumInputPorts=2
  Scope2 : Scope  NumInputPorts=2
  Scope3 : Scope
  Scope4 : Scope
  Stop Simulation : Stop
  To Workspace : ToWorkspace  VariableName=iload  SampleTime=-1
  Unit Delay2 : UnitDelay  SampleTime=-1  HasFrameUpgradeWarning=on
  Unit Delay3 : UnitDelay  SampleTime=-1  HasFrameUpgradeWarning=on
  SOC : Outport
  Draw_Pow_Lim : Outport  Port=2
  Regen_Pow_Lim : Outport  Port=3
  I batt : Outport  Port=4
  wires:
  Constant/1 -> Gain5/1
  Integrator/1 -> Gain1/1  "Watt-sec"
  Add/1 -> Compare To Constant/1, SOC/1, Scope/1, Display2/1, 1-D Lookup Table1/1, Product2/2  "batt_current_capacity_Ahr"
  Compare To Constant/1 -> Stop Simulation/1
  V/1 -> Display/1, Scope4/1, Divide/2  "normalized_ voltage"
  Gain3/1 -> Unit Delay2/1  "Power_Lim"
  Gain4/1 -> Unit Delay3/1  "Regen_Lim"
  Gain1/1 -> Scope2/2, Divide3/2  "Watt-hr"
  Divide3/1 -> Add/2
  Gain7/1 -> Add/1
  Product2/1 -> Gain4/1, Gain3/1
  Gain6/1 -> Regen_Pow_Lim/1, Scope1/2
  Constant1/1 -> Gain7/1
  Gain5/1 -> Product2/1, Divide3/1, Scope2/1  "watt-hr"
  Battery power/1 -> Divide/1, Integrator/1
  Unit Delay2/1 -> Gain/1
  Unit Delay3/1 -> Gain6/1
  Gain/1 -> Draw_Pow_Lim/1, Scope1/1
  Divide/1 -> I batt/1, To Workspace/1, Scope3/1

== system sim_battery_pack_simulink_with_EV_Load/EV model/Controller ==
  AccelCmd : Inport
  Brake : Inport  Port=2
  VehSpd : Inport  Port=3
  Draw_Lim : Inport  Port=4
  Regen_Lim : Inport  Port=5
  MtrSpd : Inport  Port=6
  Controller : Subsystem
  Scope : Scope  NumInputPorts=3
  Subsystem : Subsystem
  TrqCmd : Outport
  BrkForce : Outport  Port=2
  tag scope: BrkPrs=global, TrqCmd=global
  wires:
  Brake/1 -> Controller/2(Brake)
  [MtrSpd] -> Controller/3(MotSpd)  "mtr_spd"
  VehSpd/1 -> Controller/5(VehSpd)
  [Soc] -> Controller/4(SOC)  "batt_SOC"
  Controller/2(Brkprs) -> Scope/3, BrkForce/1, [BrkPrs]  "controller_brkforce"
  Controller/1(TrqCmd) -> Subsystem/4(controller_trqcmd), Scope/2, [TrqCmd]  "controller_trqcmd"
  AccelCmd/1 -> Controller/1(AccelCmd)
  Draw_Lim/1 -> Subsystem/1(Draw_pow_lim)
  MtrSpd/1 -> Subsystem/2(Motor_Speed)
  Regen_Lim/1 -> Subsystem/3(Regen_Pow_Lim)
  Subsystem/1(y) -> Scope/1, TrqCmd/1

== system sim_battery_pack_simulink_with_EV_Load/EV model/Driver ==
  VelFdbk : Inport
  1-D Lookup Table : Lookup_n-D  NumberOfTableDimensions=1  BreakpointsForDimension1=[T_MIDC]  Table=[V_MIDC]  InternalRulePriority=Speed  RndMeth=Simplest  InputSameDT=on
  Abs : Abs
  Clock : Clock
  Compare To Constant : simulink/Logic and Bit Operations/Compare To Constant  relop=>=  const=0  OutDataTypeStr=boolean
  Compare To Constant1 : simulink/Logic and Bit Operations/Compare To Constant  relop=<  const=0  OutDataTypeStr=boolean
  Constant1 : Constant
  Constant2 : Constant  Value=773
  Constant3 : Constant  Value=0
  Drive Cycle Source : autolibshared/Drive Cycle Source  cycleVar=FTP75  wsVar=[T_MIDC,VMIDC]  fileVar=cycleFTP75.mat  tfinal="2474  seconds, Cyclic"  cycleRepeat=on  outAccPort=off  outGearPort=off  gearList=No gear data  t_wot1=5  xdot_woto=0  xdot_wot1=30  t_wot2=20  xdot_wot2=0  t_wotend=30  srcUnit=m/s  outUnit=km/h  srcAccUnit=m/s/s  outAccUnit=m/s^2  dt=0  aMode=1  faultOption=off  velBnd=2  velBndUnit=mph  inUnit=m/s  timeBnd=1  failOption=off  stopSim=off  maxFaultCnt=10  maxFaultTime=2  maxTotFaultTime=15  traceOption=off  dtTrace=1  traceWindow=10  lastDCname=FTP75  lastOutUnit=mph  lastDT=0  lastTB=1  lastSB=2  forceCalcBound=off
      settings: SourceProductBaseCode=PW,DR,MT,UV,VE
  Gain4 : Gain  Gain=5/18
  Mod : Math  Operator=mod  SaturateOnIntegerOverflow=on
  PID Controller : slpidlib/PID Controller  Controller=PID  Form=Parallel  TimeDomain=Continuous-time  UseExternalTs=off  SampleTime=-1  IntegratorMethod=Forward Euler  FilterMethod=Forward Euler  ControllerParametersSource=internal  P=1.2  I=.1  D=.1  UseFilter=on  N=100  TunerSelectOption=Transfer Function Based (PID Tuner App)  InitialConditionSource=internal  InitialConditionForIntegrator=0  InitialConditionForFilter=0  DifferentiatorICPrevScaledInput=0  ExternalReset=none  TrackingMode=off  Kt=1  LimitOutput=on  SatLimitsSource=internal  UpperSaturationLimit=1  LowerSaturationLimit=-1  LinearizeAsGain=on  AntiWindupMode=clamping  Kb=1  POutMin=[]  POutMax=[]  IOutMin=[]  IOutMax=[]  DOutMin=[]  DOutMax=[]  NOutMin=[]  NOutMax=[]  SumOutMin=[]  SumOutMax=[]  SaturationOutMin=[]  SaturationOutMax=[]  PParamMin=[]  PParamMax=[]  IParamMin=[]  IParamMax=[]  DParamMin=[]  DParamMax=[]  NParamMin=[]  NParamMax=[]  KbParamMin=[]  KbParamMax=[]  KtParamMin=[]  KtParamMax=[]  KbOutMin=[]  KbOutMax=[]  KtOutMin=[]  KtOutMax=[]  IntegratorOutMin=[]  IntegratorOutMax=[]  FilterOutMin=[]  FilterOutMax=[]  SumI1OutMin=[]  SumI1OutMax=[]  SumI2OutMin=[]  SumI2OutMax=[]  SumI3OutMin=[]  SumI3OutMax=[]  SumI4OutMin=[]  SumI4OutMax=[]  SumDOutMin=[]  SumDOutMax=[]  DifferentiatorOutMin=[]  DifferentiatorOutMax=[]  FilterDiffOutCoefMin=[]  FilterDiffOutCoefMax=[]  ReciprocalOutMin=[]  ReciprocalOutMax=[]  SumDenOutMin=[]  SumDenOutMax=[]  SumNumOutMin=[]  SumNumOutMax=[]  DivideOutMin=[]  DivideOutMax=[]  UdiffTsProdOutMin=[]  UdiffTsProdOutMax=[]  NTsProdOutMin=[]  NTsProdOutMax=[]  UintegralTsProdOutMin=[]  UintegralTsProdOutMax=[]  UngainTsProdOutMin=[]  UngainTsProdOutMax=[]  IntegratorContinuousStateAttributes=''  IntegratorStateMustResolveToSignalObject=off  IntegratorRTWStateStorageClass=Auto  FilterContinuousStateAttributes=''  FilterStateMustResolveToSignalObject=off  FilterRTWStateStorageClass=Auto  ParallelPVariant=InternalParameters  IdealPVariant=Disabled  IVariant=InternalParameters  DVariant=InternalParameters  IntegratorVariant=Continuous  SatVariant=Enabled  AWVariant=ContClampingParallel  PCopyVariant=Disabled  TRVariant=Disabled  FdbkBlocksVariant=Forward  IdealPFdbkVariant=Disabled  SatFdbkVariant=Disabled  DerivativeFilterVariant=ContFilter  NVariant=InternalParameters  NCopyVariant=Disabled  FilterICVariant=InternalICsFilter  IntegratorICVariant=InternalICs  ExternalResetVariant=Disabled  TRSumVariant=Passthrough  SumFdbkVariant=Disabled  SumVariant=Sum_PID  TsampFilterVariant=InternalTs  TsampNgainVariant=Passthrough  TsampIntegralVariant=Passthrough  ExternalSaturationOutDataTypeStr=Inherit: Same as second input
  Product : Product
  Product1 : Product
  Scope : Scope  NumInputPorts=2
  Signal Builder1 : Subsystem  Tag=STV Subsys  Commented=on  LoadFcn=sigbuilder_block('load');  StartFcn=sigbuilder_block('start');  StopFcn=sigbuilder_block('stop');  ClipboardFcn=sigbuilder_block('clipboard');  mask(Sigbuilder block){tuvar=[0:10]}
      mask help: Simulink:masks:SigbuilderBlock_MD
      mask init:
      | if ~strcmp(get_param(bdroot(gcbh),'SimulationStatus'),'stopped') tuvar = sigbuilder_block('maskInit'); end
      settings: CopyFcn=sigbuilder_block('copy');  DeleteFcn=sigbuilder_block('delete');  ModelCloseFcn=sigbuilder_block('modelClose');  PreSaveFcn=sigbuilder_block('preSave');  PauseFcn=sigbuilder_block('pause');  ContinueFcn=sigbuilder_block('continue');  NameChangeFcn=sigbuilder_block('namechange');  OpenFcn=sigbuilder_block('open',[437.6 153 550.4 359.25 ]);  CloseFcn=sigbuilder_block('close');
      mask Display: plot(0, 0, 100, 100,[2, 2, 32, 32, 2], [68, 8, 8, 68, 68],[32, 2], [38, 38], [32, 19, 2],[53, 60, 44], [32, 17, 17, 2],[16, 16, 31, 31]);txt = getActiveGroup(gcbh);text(2, 100, txt,'verticalAlignment', 'top');
  Sum : Sum  Inputs=|+-
  AccelCmd : Outport
  DecelCmd : Outport  Port=2
  Vref : Outport  Port=3
  tag scope: RefSpd=global
  wires:
  Gain4/1 -> [RefSpd], Sum/1  "m/s"
  VelFdbk/1 -> Sum/2
  Product1/1 -> DecelCmd/1, Scope/2  "brk_cmd"
  Sum/1 -> PID Controller/1
  Compare To Constant/1 -> Product/2
  Compare To Constant1/1 -> Product1/2
  PID Controller/1 -> Compare To Constant1/1, Abs/1, Compare To Constant/1, Product/1
  Abs/1 -> Product1/1
  Clock/1 -> Mod/1
  Constant2/1 -> Mod/2
  Mod/1 -> 1-D Lookup Table/1
  1-D Lookup Table/1 -> Gain4/1, Vref/1  "acc_cmd"
  Product/1 -> AccelCmd/1, Scope/1  "acc_cmd"

== system sim_battery_pack_simulink_with_EV_Load/EV model/Motor ==
  TrqCmd : Inport
  MtrSpd : Inport  Port=2
  1-D Lookup Table : Lookup_n-D  NumberOfTableDimensions=1  BreakpointsForDimension1=M_w  Table=M_Trq  ExtrapMethod=Clip  UseLastTableValue=on  InternalRulePriority=Speed  RndMeth=Simplest  InputSameDT=on
  1-D Lookup Table1 : Lookup_n-D  NumberOfTableDimensions=1  BreakpointsForDimension1=M_w  Table=-M_Trq*0.5  ExtrapMethod=Clip  UseLastTableValue=on  InternalRulePriority=Speed  RndMeth=Simplest  InputSameDT=on
  Compare To Constant : simulink/Logic and Bit Operations/Compare To Constant  relop=>=  const=1  OutDataTypeStr=boolean
  Constant : Constant  Value=Batt_Eff
  Gain : Gain  Gain=1/Mot_Eff
  Gain1 : Gain  Gain=b
  KW : Gain  Gain=.001
  Min : MinMax  Inputs=2
  Min1 : MinMax  Function=max  Inputs=2
  Product : Product  Inputs=**
  Product1 : Product  Inputs=**
  Product2 : Product
  Scope : Scope  NumInputPorts=3
  Scope1 : Scope  NumInputPorts=3
  Scope2 : Scope  NumInputPorts=2
  Scope3 : Scope  NumInputPorts=2
  Scope4 : Scope
  Subtract : Sum  Inputs=+-
  Switch : Switch  Criteria=u2 > Threshold
  Switch1 : Switch  Criteria=u2 > Threshold
  Batt_Pow_Cons : Outport
  Mtr_trq : Outport  Port=2
  wires:
  TrqCmd/1 -> Scope3/2, Scope2/2, Min1/2, Switch1/2, Switch/2, Min/2
  Switch/1 -> Scope/1, Scope1/1, Subtract/1, Product/1
  MtrSpd/1 -> Gain1/1, Compare To Constant/1, Scope/2, Product/2, 1-D Lookup Table/1, 1-D Lookup Table1/1
  Product/1 -> Switch1/1, Product1/1, KW/1  "Mot mech power"
  1-D Lookup Table/1 -> Scope3/1, Min/1
  Product2/1 -> Scope1/2, Subtract/2
  Subtract/1 -> Scope1/3, Mtr_trq/1
  Compare To Constant/1 -> Product2/2
  Gain1/1 -> Product2/1
  Gain/1 -> Scope4/1, Batt_Pow_Cons/1  "batt_Pow"
  1-D Lookup Table1/1 -> Scope2/1, Min1/1
  Min1/1 -> Switch/3
  Min/1 -> Switch/1
  Switch1/1 -> Gain/1
  Product1/1 -> Switch1/3  "Mot mech power"
  Constant/1 -> Product1/2
  KW/1 -> Scope/3

== system sim_battery_pack_simulink_with_EV_Load/EV model/Transmission ==
  MtrTrq : Inport
  AxleSpd : Inport  Port=2
  Gain : Gain  Gain=Gr
  Gain1 : Gain  Gain=Gr
  Gain2 : Gain  Gain=Trans_Eff
  Product : Product
  Scope : Scope
  AxleTrq : Outport
  MtrSpd : Outport  Port=2
  tag scope: MtrSpd=global
  wires:
  Gain/1 -> Product/2, AxleTrq/1  "singlemotorunit_mtrtrq"
  Gain1/1 -> MtrSpd/1, [MtrSpd]  "mtr_spd_radps"
  Product/1 -> Scope/1
  Gain2/1 -> Gain/1
  AxleSpd/1 -> Gain1/1, Product/1
  MtrTrq/1 -> Gain2/1

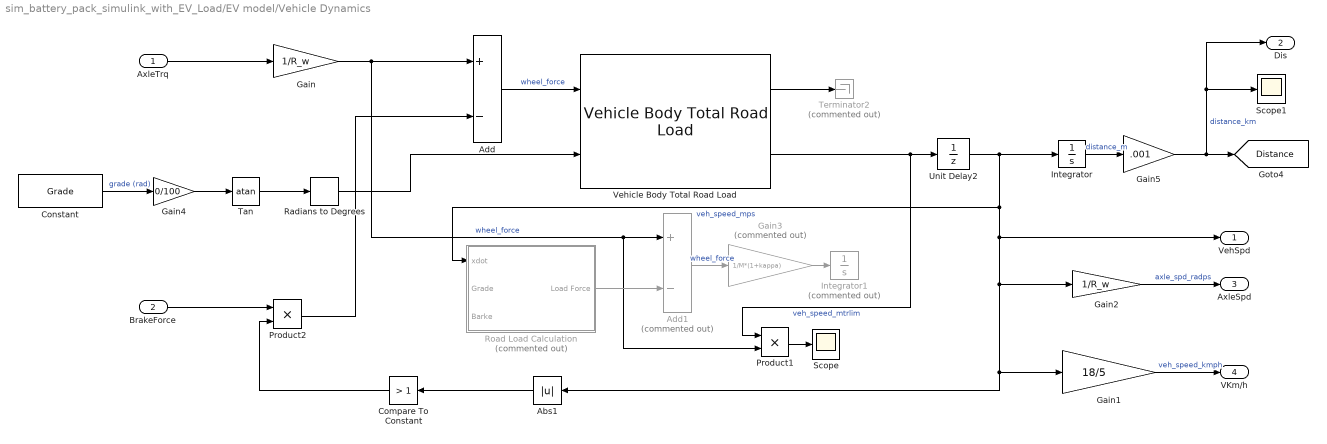
== system sim_battery_pack_simulink_with_EV_Load/EV model/Vehicle Dynamics ==
  AxleTrq : Inport
  BrakeForce : Inport  Port=2
  Abs1 : Abs
  Add : Sum  Inputs=+-
  Add1 : Sum  Commented=on  Inputs=+-
  Compare To Constant : simulink/Logic and Bit Operations/Compare To Constant  relop=>  const=1  OutDataTypeStr=boolean
  Constant : Constant  Value=Grade
  Gain : Gain  Gain=1/R_w
  Gain1 : Gain  Gain=18/5
  Gain2 : Gain  Gain=1/R_w
  Gain3 : Gain  Commented=on  Gain=1/M*(1+kappa)
  Gain4 : Gain  Gain=0/100
  Gain5 : Gain  Gain=.001
  Integrator : Integrator
  Integrator1 : Integrator  Commented=on
  Product1 : Product
  Product2 : Product
  Radians to Degrees : simulink_extras/Transformations/Radians to Degrees
  Road Load Calculation : Subsystem  Commented=on
  Scope : Scope
  Scope1 : Scope
  Tan : Trigonometry  Operator=atan
  Terminator2 : Terminator  Commented=on
  Unit Delay2 : UnitDelay  SampleTime=-1  HasFrameUpgradeWarning=on
  Vehicle Body Total Road Load : autolibshared/Vehicle Body Total Road Load  VariantControl=SL1dof  input_type=Force  aMode=1  m=M  a=M*g*mu  b=0/R_w^2  c=0.5*cd*rho*Af  g=g  x_o=0  xdot_o=0
      settings: SourceProductBaseCode=PW,DR,MT,UV,VE
  VehSpd : Outport
  Dis : Outport  Port=2
  AxleSpd : Outport  Port=3
  VKm/h : Outport  Port=4
  tag scope: Distance=global
  wires:
  Gain/1 -> Add/1, Product1/2, Add1/1  "wheel_force"
  Tan/1 -> Radians to Degrees/1
  Vehicle Body Total Road Load/1 -> Terminator2/1
  Integrator/1 -> Gain5/1  "distance_m"
  Product2/1 -> Add/2
  Gain5/1 -> Scope1/1, Dis/1, [Distance]  "distance_km"
  AxleTrq/1 -> Gain/1
  Gain2/1 -> AxleSpd/1  "axle_spd_radps"
  Gain1/1 -> VKm/h/1  "veh_speed_kmph"
  Vehicle Body Total Road Load/2 -> Unit Delay2/1, Product1/1  "veh_speed_mtrlim"
  Road Load Calculation/1(Load Force) -> Add1/2
  Add1/1 -> Gain3/1  "wheel_force"
  Gain3/1 -> Integrator1/1
  Product1/1 -> Scope/1
  Radians to Degrees/1 -> Vehicle Body Total Road Load/2
  Add/1 -> Vehicle Body Total Road Load/1  "wheel_force"
  BrakeForce/1 -> Product2/1
  Compare To Constant/1 -> Product2/2
  Abs1/1 -> Compare To Constant/1
  Constant/1 -> Gain4/1  "grade (rad)"
  Gain4/1 -> Tan/1
  Unit Delay2/1 -> VehSpd/1, Abs1/1, Gain1/1, Gain2/1, Road Load Calculation/1(xdot), Integrator/1  "veh_speed_mps"

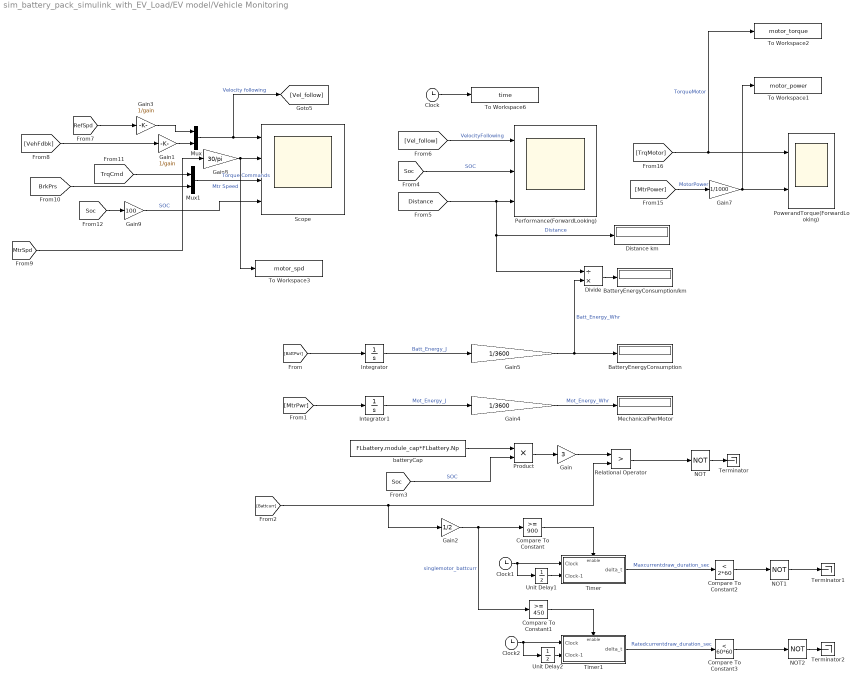
== system sim_battery_pack_simulink_with_EV_Load/EV model/Vehicle Monitoring ==
  BatteryEnergyConsumption : Display
  BatteryEnergyConsumption/km : Display
  Clock : Clock
  Clock1 : Clock
  Clock2 : Clock
  Compare To Constant : simulink/Logic and Bit Operations/Compare To Constant  relop=>=  const=900  OutDataTypeStr=boolean
  Compare To Constant1 : simulink/Logic and Bit Operations/Compare To Constant  relop=>=  const=450  OutDataTypeStr=boolean
  Compare To Constant2 : simulink/Logic and Bit Operations/Compare To Constant  relop=<  const=2*60  OutDataTypeStr=boolean
  Compare To Constant3 : simulink/Logic and Bit Operations/Compare To Constant  relop=<  const=60*60  OutDataTypeStr=boolean
  Distance km : Display
  Divide : Product  Inputs=/*
  Gain : Gain  Gain=3
  Gain1 : Gain  Gain=1/gain
  Gain2 : Gain  Gain=1/2
  Gain3 : Gain  Gain=1/gain
  Gain4 : Gain  Gain=1/3600
  Gain5 : Gain  Gain=1/3600
  Gain7 : Gain  Gain=1/1000
  Gain8 : Gain  Gain=30/pi
  Gain9 : Gain  Gain=100
  Integrator : Integrator
  Integrator1 : Integrator
  MechanicalPwrMotor : Display
  Mux : Mux  Inputs=2
  Mux1 : Mux  Inputs=2
  NOT : Logic  Operator=NOT  IconShape=distinctive  AllPortsSameDT=off  OutDataTypeStr=boolean
  NOT1 : Logic  Operator=NOT  IconShape=distinctive  AllPortsSameDT=off  OutDataTypeStr=boolean
  NOT2 : Logic  Operator=NOT  IconShape=distinctive  AllPortsSameDT=off  OutDataTypeStr=boolean
  Performance(ForwardLooking) : Scope  NumInputPorts=3
  PowerandTorque(ForwardLooking) : Scope  NumInputPorts=2
  Product : Product
  Relational Operator : RelationalOperator  Operator=>  OutDataTypeStr=boolean  RndMeth=Simplest
  Scope : Scope  NumInputPorts=4
  Terminator : Terminator
  Terminator1 : Terminator
  Terminator2 : Terminator
  Timer : Subsystem  TreatAsAtomicUnit=on
  Timer1 : Subsystem  TreatAsAtomicUnit=on
  To Workspace1 : ToWorkspace  VariableName=motor_power  SampleTime=-1
      settings: Save2DSignal=2-D array (concatenate along first dimension)
  To Workspace2 : ToWorkspace  VariableName=motor_torque  SampleTime=-1
      settings: Save2DSignal=2-D array (concatenate along first dimension)
  To Workspace3 : ToWorkspace  VariableName=motor_spd  SampleTime=-1
      settings: Save2DSignal=2-D array (concatenate along first dimension)
  To Workspace6 : ToWorkspace  VariableName=time  SampleTime=-1
      settings: Save2DSignal=2-D array (concatenate along first dimension)
  Unit Delay1 : UnitDelay  SampleTime=-1  HasFrameUpgradeWarning=on
  Unit Delay2 : UnitDelay  SampleTime=-1  HasFrameUpgradeWarning=on
  batteryCap : Constant  Value=FLbattery.module_cap*FLbattery.Np
  wires:
  Gain1/1 -> Mux/2
  Mux/1 -> [Vel_follow], Scope/1  "Velocity following"
  Clock/1 -> To Workspace6/1
  [Vel_follow] -> Performance(ForwardLooking)/1  "VelocityFollowing"
  [BrkPrs] -> Mux1/2
  [TrqMotor] -> To Workspace2/1, PowerandTorque(ForwardLooking)/1  "TorqueMotor"
  [RefSpd] -> Gain3/1
  [MtrSpd] -> Gain8/1
  Gain8/1 -> To Workspace3/1, Scope/2  "Mtr Speed"
  [TrqCmd] -> Mux1/1
  [MtrPower] -> Gain7/1  "MotorPower"
  Gain3/1 -> Mux/1
  Mux1/1 -> Scope/3  "Torque Commands"
  [Soc] -> Gain9/1
  [Soc] -> Performance(ForwardLooking)/2  "SOC"
  [Distance] -> Divide/1, Distance km/1, Performance(ForwardLooking)/3  "Distance"
  Gain7/1 -> To Workspace1/1, PowerandTorque(ForwardLooking)/2
  [VehFdbk] -> Gain1/1
  Gain9/1 -> Scope/4  "SOC"
  [BattPwr] -> Integrator/1
  Integrator/1 -> Gain5/1  "Batt_Energy_J"
  Gain5/1 -> Divide/2, BatteryEnergyConsumption/1  "Batt_Energy_Whr"
  Divide/1 -> BatteryEnergyConsumption/km/1
  [MtrPwr] -> Integrator1/1
  Integrator1/1 -> Gain4/1  "Mot_Energy_J"
  Gain4/1 -> MechanicalPwrMotor/1  "Mot_Energy_Whr"
  [Battcurr] -> Relational Operator/2, Gain2/1
  [Soc] -> Product/2  "SOC"
  batteryCap/1 -> Product/1
  Product/1 -> Gain/1
  Gain/1 -> Relational Operator/1
  Relational Operator/1 -> NOT/1
  Clock1/1 -> Unit Delay1/1, Timer/1(Clock)
  Unit Delay1/1 -> Timer/2(Clock-1)
  Compare To Constant/1 -> Timer/Enable
  Gain2/1 -> Compare To Constant1/1, Compare To Constant/1  "singlemotor_battcurr"
  Timer/1(delta_t) -> Compare To Constant2/1  "Maxcurrentdraw_duration_sec"
  Compare To Constant2/1 -> NOT1/1
  Unit Delay2/1 -> Timer1/2(Clock-1)
  Clock2/1 -> Unit Delay2/1, Timer1/1(Clock)
  Timer1/1(delta_t) -> Compare To Constant3/1  "Ratedcurrentdraw_duration_sec"
  Compare To Constant1/1 -> Timer1/Enable
  Compare To Constant3/1 -> NOT2/1
  NOT/1 -> Terminator/1
  NOT1/1 -> Terminator1/1
  NOT2/1 -> Terminator2/1

== system sim_battery_pack_simulink_with_EV_Load/SCM1/cell1 ==
  ik1 : Inport
  Constant : Constant  Value=R0
  Constant1 : Constant  Value=dt
  Constant2 : Constant  Value=T
  States : Scope  NumInputPorts=2
  Unit Delay : UnitDelay  InitialCondition=Z0(1,1)  SampleTime=-1  HasFrameUpgradeWarning=on
  Unit Delay1 : UnitDelay  SampleTime=-1  HasFrameUpgradeWarning=on
  Voltage : Scope  NumInputPorts=2
  cell_model : MATLAB Function  TreatAsAtomicUnit=on
  V1 : Outport
  Z1 : Outport  Port=2
  irc1 : Outport  Port=3
  wires:
  cell_model/4(OCV) -> Voltage/2
  ik1/1 -> cell_model/6(ik)
  cell_model/3(zkc) -> Z1/1, Unit Delay/1, States/1
  cell_model/1(vk) -> V1/1, Voltage/1
  Constant1/1 -> cell_model/2(deltaT)
  Constant2/1 -> cell_model/1(T)
  Unit Delay/1 -> cell_model/4(zkp)
  cell_model/2(irkc) -> irc1/1, Unit Delay1/1, States/2
  Unit Delay1/1 -> cell_model/5(irkp)
  Constant/1 -> cell_model/3(iR0)

== system sim_battery_pack_simulink_with_EV_Load/SCM1/cell10 ==
  ik1 : Inport
  Constant : Constant  Value=R0
  Constant1 : Constant  Value=dt
  Constant2 : Constant  Value=T
  States : Scope  NumInputPorts=2
  Unit Delay : UnitDelay  InitialCondition=Z0(10,1)  SampleTime=-1  HasFrameUpgradeWarning=on
  Unit Delay1 : UnitDelay  SampleTime=-1  HasFrameUpgradeWarning=on
  Voltage : Scope  NumInputPorts=2
  cell_model : MATLAB Function  TreatAsAtomicUnit=on
  V1 : Outport
  Z1 : Outport  Port=2
  irc1 : Outport  Port=3
  wires:
  cell_model/4(OCV) -> Voltage/2
  ik1/1 -> cell_model/6(ik)
  cell_model/3(zkc) -> Z1/1, Unit Delay/1, States/1
  cell_model/1(vk) -> V1/1, Voltage/1
  Constant1/1 -> cell_model/2(deltaT)
  Constant2/1 -> cell_model/1(T)
  Unit Delay/1 -> cell_model/4(zkp)
  cell_model/2(irkc) -> irc1/1, Unit Delay1/1, States/2
  Unit Delay1/1 -> cell_model/5(irkp)
  Constant/1 -> cell_model/3(iR0)

== system sim_battery_pack_simulink_with_EV_Load/SCM1/cell11 ==
  ik1 : Inport
  Constant : Constant  Value=R0
  Constant1 : Constant  Value=dt
  Constant2 : Constant  Value=T
  States : Scope  NumInputPorts=2
  Unit Delay : UnitDelay  InitialCondition=Z0(11,1)  SampleTime=-1  HasFrameUpgradeWarning=on
  Unit Delay1 : UnitDelay  SampleTime=-1  HasFrameUpgradeWarning=on
  Voltage : Scope  NumInputPorts=2
  cell_model : MATLAB Function  TreatAsAtomicUnit=on
  V1 : Outport
  Z1 : Outport  Port=2
  irc1 : Outport  Port=3
  wires:
  Constant/1 -> cell_model/3(iR0)
  Unit Delay1/1 -> cell_model/5(irkp)
  cell_model/2(irkc) -> States/2, Unit Delay1/1, irc1/1
  Unit Delay/1 -> cell_model/4(zkp)
  Constant2/1 -> cell_model/1(T)
  Constant1/1 -> cell_model/2(deltaT)
  cell_model/1(vk) -> Voltage/1, V1/1
  cell_model/3(zkc) -> States/1, Unit Delay/1, Z1/1
  ik1/1 -> cell_model/6(ik)
  cell_model/4(OCV) -> Voltage/2

== system sim_battery_pack_simulink_with_EV_Load/SCM1/cell12 ==
  ik1 : Inport
  Constant : Constant  Value=R0
  Constant1 : Constant  Value=dt
  Constant2 : Constant  Value=T
  States : Scope  NumInputPorts=2
  Unit Delay : UnitDelay  InitialCondition=Z0(12,1)  SampleTime=-1  HasFrameUpgradeWarning=on
  Unit Delay1 : UnitDelay  SampleTime=-1  HasFrameUpgradeWarning=on
  Voltage : Scope  NumInputPorts=2
  cell_model : MATLAB Function  TreatAsAtomicUnit=on
  V1 : Outport
  Z1 : Outport  Port=2
  irc1 : Outport  Port=3
  wires:
  Constant/1 -> cell_model/3(iR0)
  Unit Delay1/1 -> cell_model/5(irkp)
  cell_model/2(irkc) -> States/2, Unit Delay1/1, irc1/1
  Unit Delay/1 -> cell_model/4(zkp)
  Constant2/1 -> cell_model/1(T)
  Constant1/1 -> cell_model/2(deltaT)
  cell_model/1(vk) -> Voltage/1, V1/1
  cell_model/3(zkc) -> States/1, Unit Delay/1, Z1/1
  ik1/1 -> cell_model/6(ik)
  cell_model/4(OCV) -> Voltage/2

== system sim_battery_pack_simulink_with_EV_Load/SCM1/cell2 ==
  ik1 : Inport
  Constant : Constant  Value=R0
  Constant1 : Constant  Value=dt
  Constant2 : Constant  Value=T
  States : Scope  NumInputPorts=2
  Unit Delay : UnitDelay  InitialCondition=Z0(2,1)  SampleTime=-1  HasFrameUpgradeWarning=on
  Unit Delay1 : UnitDelay  SampleTime=-1  HasFrameUpgradeWarning=on
  Voltage : Scope  NumInputPorts=2
  cell_model : MATLAB Function  TreatAsAtomicUnit=on
  V1 : Outport
  Z1 : Outport  Port=2
  irc1 : Outport  Port=3
  wires:
  cell_model/4(OCV) -> Voltage/2
  ik1/1 -> cell_model/6(ik)
  cell_model/3(zkc) -> Z1/1, Unit Delay/1, States/1
  cell_model/1(vk) -> V1/1, Voltage/1
  Constant1/1 -> cell_model/2(deltaT)
  Constant2/1 -> cell_model/1(T)
  Unit Delay/1 -> cell_model/4(zkp)
  cell_model/2(irkc) -> irc1/1, Unit Delay1/1, States/2
  Unit Delay1/1 -> cell_model/5(irkp)
  Constant/1 -> cell_model/3(iR0)

== system sim_battery_pack_simulink_with_EV_Load/SCM1/cell3 ==
  ik1 : Inport
  Constant : Constant  Value=R0
  Constant1 : Constant  Value=dt
  Constant2 : Constant  Value=T
  States : Scope  NumInputPorts=2
  Unit Delay : UnitDelay  InitialCondition=Z0(3,1)  SampleTime=-1  HasFrameUpgradeWarning=on
  Unit Delay1 : UnitDelay  SampleTime=-1  HasFrameUpgradeWarning=on
  Voltage : Scope  NumInputPorts=2
  cell_model : MATLAB Function  TreatAsAtomicUnit=on
  V1 : Outport
  Z1 : Outport  Port=2
  irc1 : Outport  Port=3
  wires:
  Constant/1 -> cell_model/3(iR0)
  Unit Delay1/1 -> cell_model/5(irkp)
  cell_model/2(irkc) -> States/2, Unit Delay1/1, irc1/1
  Unit Delay/1 -> cell_model/4(zkp)
  Constant2/1 -> cell_model/1(T)
  Constant1/1 -> cell_model/2(deltaT)
  cell_model/1(vk) -> Voltage/1, V1/1
  cell_model/3(zkc) -> States/1, Unit Delay/1, Z1/1
  ik1/1 -> cell_model/6(ik)
  cell_model/4(OCV) -> Voltage/2
